simulink model "Modello_definitivo"  (Simulink 9.2)
settings: Solver=ode45  StartTime=0*24*3600  StopTime=365*24*3600  MaxStep=3600  RelTol=1e-3  SampleTimeConstraint=Specified  EnableMultiTasking=on
undefined symbols (not defined in the file or in its folder): T_s_in
libraries: simulink x1
(part 1 of 2)
settings Model: Creator=Matteo  LastModifiedBy=don-g
settings SolverCC: ZeroCrossControl=DisableAll
settings OptimizationCC: ExpressionDepthLimit=2147483647  InitFltsAndDblsToZero=on
settings DebuggingCC: SolverPrmCheckMsg=warning
settings SFSimCC: SimUseLocalCustomCode=on
settings RTWCC: RTWUseLocalCustomCode=on
settings GRTTargetCC: GeneratePreprocessorConditionals=Use local settings
settings ConfigComp: CovExternalEMLEnable=on

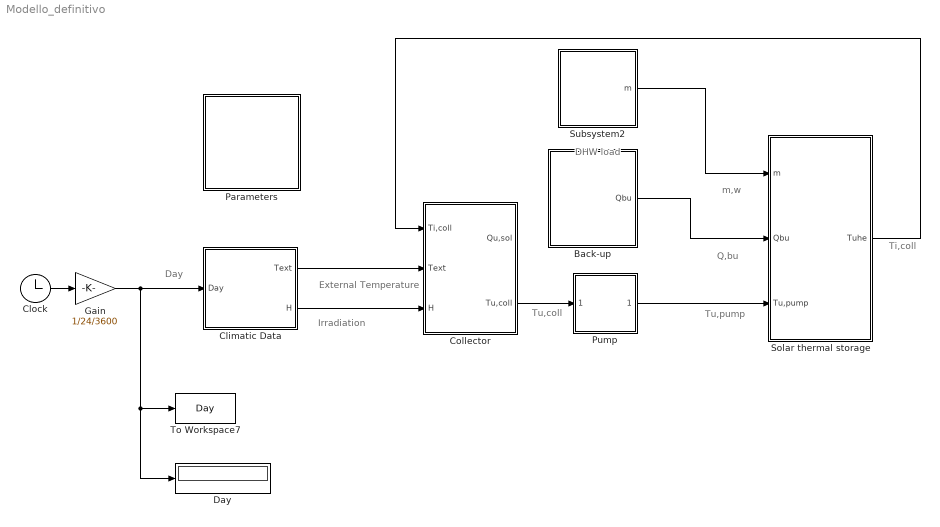
== system Modello_definitivo ==
  note: Q,bu
  note: m,w
  note: Day
  note: Irradiation
  note: External Temperature
  note: Tu,coll
  note: DHW load
  note: Tu,pump
  note: Ti,coll
  Back-up : Subsystem
      mask Display: image(imread('caldaia.jpg'))
  Climatic Data : Subsystem
      mask Display: image(imread('sole.jpg'))
  Clock : Clock
  Collector : Subsystem
      mask Display: image(imread('collettore.jpg'))
  Day : Display
  Gain : Gain  Gain=1/24/3600  SaturateOnIntegerOverflow=on  OutDataTypeStr=Inherit: Same as input  ParamDataTypeStr=Inherit: Same as input
  Parameters : Subsystem  mask{Gamma=0, Rho=0.2, Lat=44.48, Beta=0.01, Eta0=0.959, a1=8.91, a2=0.047, Nc=1, Aap=2.31, m_brine=0.010, Cp_brine=3900, L=1.7, Eta_pump=0.8, Eta_el=0.95, H_pressure=50000, Pump_power=65, Rho_brine=1037, T_room=20, BU_power=2000, Rho_water=1000, Cp_water=4186, U_s=1, T_s_in=45, D_s=0.6, V_s=168, H_s=0.99, UA_s_ex=167, T_s_max=90, A_s_ex=1.8, U_s_ex=1.1, T_DHW=45, S_u=200, T_acq=15}
      mask prompts: Gamma "Azimuth (°)"; Rho "Albedo"; Lat "Latitude (°)"; Beta "Tilt (°)"; Eta0 "Optical efficiency"; a1 "First order coefficient"; a2 "Second order coefficient"; Nc "Number of collectors"; Aap "Absorber area (m2)"; m_brine "Flow rate per surface area (kg/s*m2)"; Cp_brine "Cp brine (J/kgK)"; L "Collector liquid volume (lt)"; Eta_pump "Pump efficiency"; Eta_el "Electrical efficiency"; H_pressure "Head pressure (Pa)"; Pump_power "Pump power (W)"; Rho_brine "Brine density (kg/m3)"; T_room "Room temperature (°C)"; BU_power "Back-up power (W)"; Rho_water "Water density (kg/m3)"; Cp_water "Cp water (J/kgK)"; U_s "Storage U (W/m2K)"; T_s_in "Initial storage temperature (°C)"; D_s "Storage diameter (m)"; V_s "Storage volume (lt)"; H_s "Storage height (m)"; UA_s_ex "Solar exchanger UA (W/K)"; T_s_max "Maximum storage temperature (°C)"; A_s_ex "Heat exchanger area (m2)"; U_s_ex "U-value heat exchanger (W/m2K)"; T_DHW "DHW temperature (°C)"; S_u "Building energetic surface (m2)"; T_acq "Aqueduct temperature (°C)"
      mask Display: image(imread('images.jpg'))
  Pump : Subsystem
      mask Display: image(imread('pompa.jpg'))
  Solar thermal storage : Subsystem
      mask Display: image(imread('prova.jpg'))
  Subsystem2 : Subsystem
      mask Display: image(imread('casa.jpg'))
  To Workspace7 : ToWorkspace  VariableName=Day  SampleTime=[3600 0]
  wires:
  Gain/1 -> Climatic Data/1(Day), Day/1, To Workspace7/1
  Clock/1 -> Gain/1
  Climatic Data/1(Text) -> Collector/2(Text)
  Climatic Data/2(H) -> Collector/3(H)
  Collector/2(Tu,coll) -> Pump/1(Tu,coll)
  Subsystem2/1(m) -> Solar thermal storage/1(m)
  Pump/1(Tu,pump) -> Solar thermal storage/3(Tu,pump)
  Solar thermal storage/1(Tuhe) -> Collector/1(Ti,coll)
  Back-up/1(Qbu) -> Solar thermal storage/2(Qbu)

== system Modello_definitivo/Back-up ==
  Add1 : Sum  Inputs=-+
  Back-up energy [MJ] : Display
  Back-up energy [kWh] : Display
  Integral Block : Subsystem
  Product3 : Product  Inputs=**  SaturateOnIntegerOverflow=on  OutDataTypeStr=Inherit: Same as first input
  Prova back-up : Subsystem
  Relay : Relay  OnSwitchValue=0  OffSwitchValue=-5
  Scope2 : Scope
  To Workspace1 : ToWorkspace  VariableName=Ebu  SampleTime=[3600 0]
  To Workspace6 : ToWorkspace  VariableName=Qbu  SampleTime=[3600 0]
  Qbu : Outport
  tag scope: Ebu_kWh=global, Qbu=global
  wires:
  [T_DHW] -> Add1/2
  [T3] -> Add1/1
  Add1/1 -> Relay/1, Scope2/1
  Relay/1 -> Product3/2
  [BU_power] -> Product3/1
  Product3/1 -> Integral Block/1(Watt), [Qbu], To Workspace6/1, Qbu/1
  Integral Block/1(MJ) -> Back-up energy [MJ]/1
  Integral Block/2(kWh) -> [Ebu_kWh], Back-up energy [kWh]/1, To Workspace1/1

== system Modello_definitivo/Climatic Data ==
  Day : Inport
  Day Length [h] : Display
  From Workspace : FromWorkspace  VariableName=Irraggiamento_Globale_Wh  SampleTime=0
  From Workspace1 : FromWorkspace  VariableName=Temperature  SampleTime=0
  Mux4 : Mux  Inputs=2
  Scope16 : Scope
  Scope6 : Scope
  To Workspace2 : ToWorkspace  VariableName=Text  SampleTime=[3600 0]
  irraggiamento : Subsystem
  Text : Outport  SampleTime=[3600 0]
  H : Outport  Port=2
  tag scope: H=global
  wires:
  From Workspace1/1 -> Scope16/1, Text/1, To Workspace2/1
  From Workspace/1 -> Mux4/2, Scope6/1
  irraggiamento/2(Day Length) -> Day Length [h]/1
  irraggiamento/1(H) -> H/1, [H]
  Mux4/1 -> irraggiamento/1(Climatic Data Input)
  Day/1 -> Mux4/1

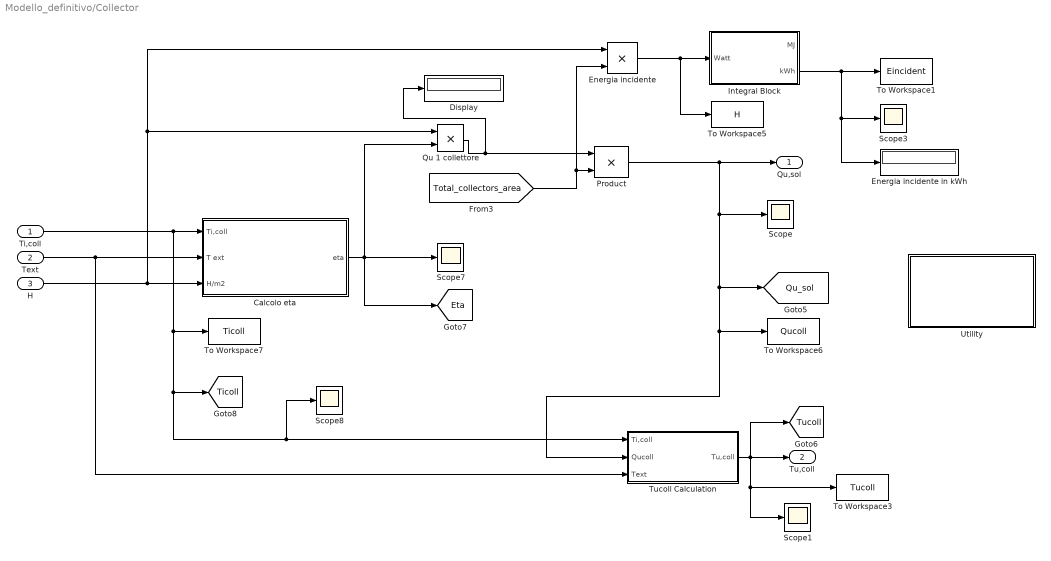
== system Modello_definitivo/Collector ==
  Ti,coll : Inport
  Text : Inport  Port=2
  H : Inport  Port=3
  Calcolo eta : Subsystem
  Display : Display
  Energia incidente : Product  RndMeth=Zero
  Energia incidente in kWh : Display
  Integral Block : Subsystem
  Product : Product  RndMeth=Zero
  Qu 1 collettore : Product  RndMeth=Zero
  Scope{,1,3,7..8} (5 alike) : Scope
  To Workspace1 : ToWorkspace  VariableName=Eincident  SampleTime=[3600 0]
  To Workspace3 : ToWorkspace  VariableName=Tucoll  SampleTime=[3600 0]
  To Workspace5 : ToWorkspace  VariableName=H  SampleTime=[3600 0]
  To Workspace6 : ToWorkspace  VariableName=Qucoll  SampleTime=[3600 0]
  To Workspace7 : ToWorkspace  VariableName=Ticoll  SampleTime=[3600 0]
  Tucoll Calculation : Subsystem
  Utility : Subsystem
  Qu,sol : Outport
  Tu,coll : Outport  Port=2
  tag scope: Eta=global, Qu_sol=global, Ticoll=global, Tucoll=global
  wires:
  H/1 -> Calcolo eta/3(H/m2), Qu 1 collettore/1, Energia incidente/1
  Text/1 -> Calcolo eta/2(T ext), Tucoll Calculation/3(Text)
  Calcolo eta/1(eta) -> [Eta], Qu 1 collettore/2, Scope7/1
  Qu 1 collettore/1 -> Product/1, Display/1
  Tucoll Calculation/1(Tu,coll) -> Tu,coll/1, Scope1/1, To Workspace3/1, [Tucoll]
  Energia incidente/1 -> Integral Block/1(Watt), To Workspace5/1
  Product/1 -> Qu,sol/1, [Qu_sol], To Workspace6/1, Tucoll Calculation/2(Qucoll), Scope/1
  Ti,coll/1 -> [Ticoll], Tucoll Calculation/1(Ti,coll), Scope8/1, To Workspace7/1, Calcolo eta/1(Ti,coll)
  Integral Block/2(kWh) -> To Workspace1/1, Scope3/1, Energia incidente in kWh/1
  [Total_collectors_area] -> Product/2, Energia incidente/2

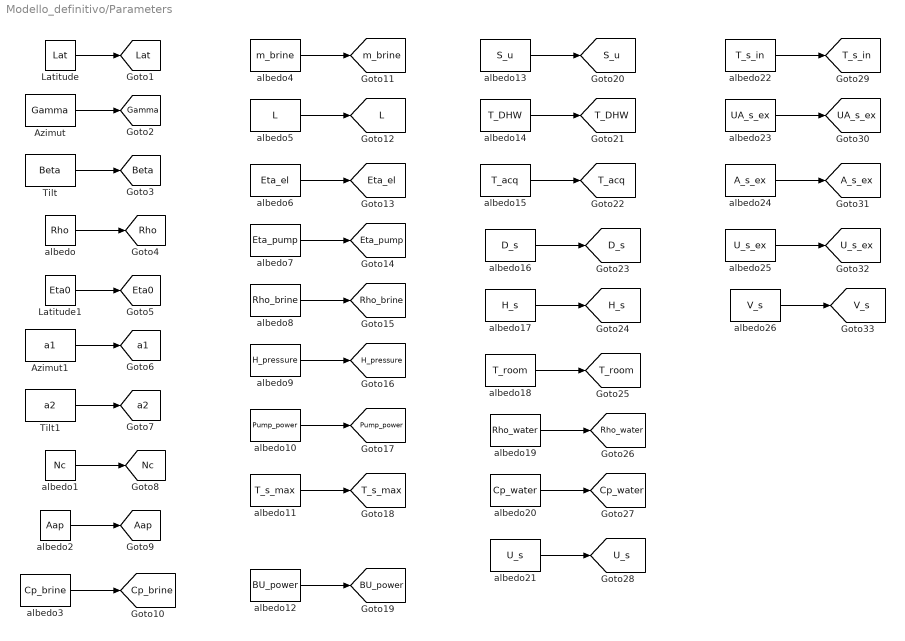
== system Modello_definitivo/Parameters ==
  Azimut : Constant  Value=Gamma
  Azimut1 : Constant  Value=a1
  Latitude : Constant  Value=Lat
  Latitude1 : Constant  Value=Eta0
  Tilt : Constant  Value=Beta
  Tilt1 : Constant  Value=a2
  albedo : Constant  Value=Rho
  albedo1 : Constant  Value=Nc
  albedo10 : Constant  Value=Pump_power
  albedo11 : Constant  Value=T_s_max
  albedo12 : Constant  Value=BU_power
  albedo13 : Constant  Value=S_u
  albedo14 : Constant  Value=T_DHW
  albedo15 : Constant  Value=T_acq
  albedo16 : Constant  Value=D_s
  albedo17 : Constant  Value=H_s
  albedo18 : Constant  Value=T_room
  albedo19 : Constant  Value=Rho_water
  albedo2 : Constant  Value=Aap
  albedo20 : Constant  Value=Cp_water
  albedo21 : Constant  Value=U_s
  albedo22 : Constant  Value=T_s_in
  albedo23 : Constant  Value=UA_s_ex
  albedo24 : Constant  Value=A_s_ex
  albedo25 : Constant  Value=U_s_ex
  albedo26 : Constant  Value=V_s
  albedo3 : Constant  Value=Cp_brine
  albedo4 : Constant  Value=m_brine
  albedo5 : Constant  Value=L
  albedo6 : Constant  Value=Eta_el
  albedo7 : Constant  Value=Eta_pump
  albedo8 : Constant  Value=Rho_brine
  albedo9 : Constant  Value=H_pressure
  tag scope: A_s_ex=global, Aap=global, BU_power=global, Beta=global, Cp_brine=global, Cp_water=global, D_s=global, Eta0=global, Eta_el=global, Eta_pump=global, Gamma=global, H_pressure=global, H_s=global, L=global, Lat=global, Nc=global, Pump_power=global, Rho=global, Rho_brine=global, Rho_water=global, S_u=global, T_DHW=global, T_acq=global, T_room=global, T_s_in=global, T_s_max=global, UA_s_ex=global, U_s=global, U_s_ex=global, V_s=global, a1=global, a2=global, m_brine=global
  wires:
  Latitude/1 -> [Lat]
  Azimut/1 -> [Gamma]
  Tilt/1 -> [Beta]
  albedo/1 -> [Rho]
  Latitude1/1 -> [Eta0]
  Azimut1/1 -> [a1]
  Tilt1/1 -> [a2]
  albedo1/1 -> [Nc]
  albedo2/1 -> [Aap]
  albedo3/1 -> [Cp_brine]
  albedo4/1 -> [m_brine]
  albedo5/1 -> [L]
  albedo6/1 -> [Eta_el]
  albedo7/1 -> [Eta_pump]
  albedo8/1 -> [Rho_brine]
  albedo9/1 -> [H_pressure]
  albedo10/1 -> [Pump_power]
  albedo11/1 -> [T_s_max]
  albedo12/1 -> [BU_power]
  albedo13/1 -> [S_u]
  albedo14/1 -> [T_DHW]
  albedo15/1 -> [T_acq]
  albedo16/1 -> [D_s]
  albedo17/1 -> [H_s]
  albedo18/1 -> [T_room]
  albedo19/1 -> [Rho_water]
  albedo20/1 -> [Cp_water]
  albedo21/1 -> [U_s]
  albedo22/1 -> [T_s_in]
  albedo23/1 -> [UA_s_ex]
  albedo24/1 -> [A_s_ex]
  albedo25/1 -> [U_s_ex]
  albedo26/1 -> [V_s]

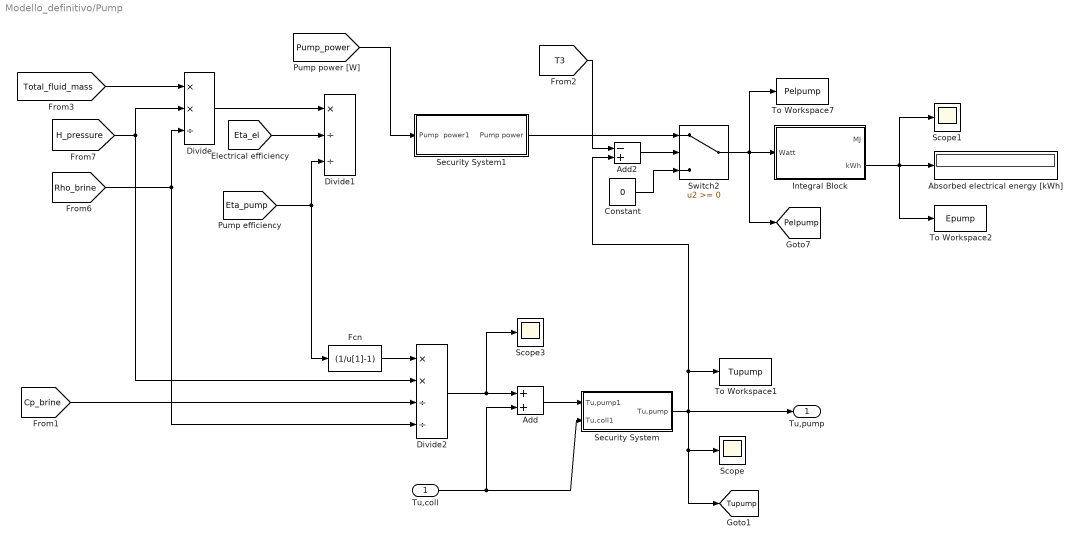
== system Modello_definitivo/Pump ==
  Tu,coll : Inport
  Absorbed electrical energy [kWh] : Display
  Add : Sum
  Add2 : Sum  Inputs=-+
  Constant : Constant  Value=0
  Divide : Product  Inputs=**/
  Divide1 : Product  Inputs=*//
  Divide2 : Product  Inputs=**//
  Fcn : Fcn  Expr=(1/u[1]-1)
  Integral Block : Subsystem
  Scope : Scope
  Scope1 : Scope
  Scope3 : Scope
  Security System : Subsystem
  Security System1 : Subsystem
  Switch2 : Switch  ZeroCross=off
  To Workspace1 : ToWorkspace  VariableName=Tupump  SampleTime=[3600 0]
  To Workspace2 : ToWorkspace  VariableName=Epump  SampleTime=[3600 0]
  To Workspace7 : ToWorkspace  VariableName=Pelpump  SampleTime=[3600 0]
  Tu,pump : Outport
  tag scope: Pelpump=global, Tupump=global
  wires:
  [Total_fluid_mass] -> Divide/1
  [H_pressure] -> Divide/2, Divide2/2
  [Rho_brine] -> Divide/3, Divide2/4
  Divide/1 -> Divide1/1
  [Eta_pump] -> Fcn/1, Divide1/3
  Fcn/1 -> Divide2/1
  Divide2/1 -> Add/1, Scope3/1
  Tu,coll/1 -> Security System/2(Tu,coll1), Add/2
  [Cp_brine] -> Divide2/3
  Integral Block/2(kWh) -> Absorbed electrical energy [kWh]/1, Scope1/1, To Workspace2/1
  Add/1 -> Security System/1(Tu,pump1)
  Security System/1(Tu,pump) -> To Workspace1/1, Add2/2, Scope/1, [Tupump], Tu,pump/1
  [Eta_el] -> Divide1/2
  [Pump_power] -> Security System1/1(Pump  power1)
  Security System1/1(Pump power) -> Switch2/1
  Add2/1 -> Switch2/2
  [T3] -> Add2/1
  Switch2/1 -> To Workspace7/1, [Pelpump], Integral Block/1(Watt)
  Constant/1 -> Switch2/3

== system Modello_definitivo/Solar thermal storage ==
  note: V[m3]
  m : Inport
  Qbu : Inport  Port=2
  Tu,pump : Inport  Port=3
  Divide : Product  Inputs=*/
  Lower part 3 : Subsystem
  Tuhe : Outport
  tag scope: m=global
  wires:
  [V_s] -> Divide/1
  Divide/1 -> Lower part 3/1(V)
  [Rho_water] -> Divide/2
  Lower part 3/2(Tuhe) -> Tuhe/1
  Tu,pump/1 -> Lower part 3/2(Tupump)
  Qbu/1 -> Lower part 3/3(Qbu)
  m/1 -> [m]

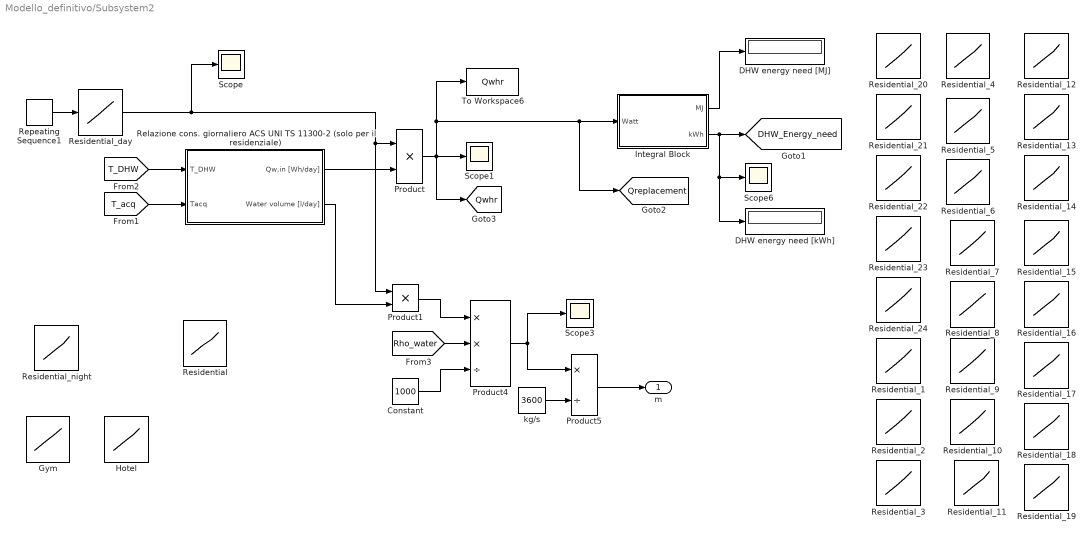
== system Modello_definitivo/Subsystem2 ==
  Constant : Constant  Value=1000
  DHW energy need [MJ] : Display
      settings: Format=bank
  DHW energy need [kWh] : Display
  Gym : Lookup  InputValues=[0*3600 1*3600 2*3600 3*3600 4*3600 5*3600 6*3600 7*3600 8*3600 9*3600 10*3600 11*3600 12*3600 13*3600 14*3600 15*3600 16*3600 17*3600 18*3600 19*3600 20*3600 21*3600 22*3600 23*3600 24*3600]  Table=[0.028 0 0 0 0 0 0 0 0.007 0.025 0.025 0.028 0.139 0.139 0.139 0.028 0.028 0.028 0.139 0.139 0.028 0.139 0.0139 0.0139 0.028]  SaturateOnIntegerOverflow=on
  Hotel : Lookup  InputValues=[0*3600 6.5*3600 6.5*3600 9.5*3600 9.5*3600 18.5*3600 18.5*3600 21*3600 21*3600 24*3600]  SaturateOnIntegerOverflow=on
  Integral Block : Subsystem
  Product : Product  SaturateOnIntegerOverflow=on  OutDataTypeStr=Inherit: Same as first input
  Product1 : Product  SaturateOnIntegerOverflow=on  OutDataTypeStr=Inherit: Same as first input
  Product4 : Product  Inputs=**/  SaturateOnIntegerOverflow=on  OutDataTypeStr=Inherit: Same as first input
  Product5 : Product  Inputs=*/  SaturateOnIntegerOverflow=on  OutDataTypeStr=Inherit: Same as first input
  Relazione cons. giornaliero ACS UNI TS 11300-2 (solo per il residenziale) : Subsystem
  Repeating Sequence1 : simulink/Sources/Repeating Sequence  rep_seq_t=[0 24*3600]  rep_seq_y=[0 24*3600]
  Residential : Lookup  InputValues=[0*3600 1*3600 2*3600 3*3600 4*3600 5*3600 6*3600 7*3600 8*3600 9*3600 10*3600 11*3600 12*3600 13*3600 14*3600 15*3600 16*3600 17*3600 18*3600 19*3600 20*3600 21*3600 22*3600 23*3600 24*3600]  Table=[0 0.025 0.028 0.028 0 0 0 0.139 0.139 0.139 0.028 0.028 0.028 0.028 0.007 0.007 0.007 0.007 0.139 0.139 0.028 0.028 0.028 0 0]  SaturateOnIntegerOverflow=on
  Residential_1 : Lookup  InputValues=[0,3600,7200,10800,14400,18000,21600,25200,28800,32400,36000,39600,43200,46800,50400,54000,57600,61200,64800,68400,72000,75600,79200,82800,86400]  Table=[0.2,0.2,0.2,0,0,0,0,0,0,0,0,0,0,0,0,0,0,0,0,0,0,0,0.2,0.2,0.2]  SaturateOnIntegerOverflow=on
  Residential_10 : Lookup  InputValues=[0,3600,7200,10800,14400,18000,21600,25200,28800,32400,36000,39600,43200,46800,50400,54000,57600,61200,64800,68400,72000,75600,79200,82800,86400]  Table=[0,0,0,0,0,0,0,0.2,0.2,0.2,0.2,0.2,0,0,0,0,0,0,0,0,0,0,0,0,0]  SaturateOnIntegerOverflow=on
  Residential_11 : Lookup  InputValues=[0,3600,7200,10800,14400,18000,21600,25200,28800,32400,36000,39600,43200,46800,50400,54000,57600,61200,64800,68400,72000,75600,79200,82800,86400]  Table=[0,0,0,0,0,0,0,0,0.2,0.2,0.2,0.2,0.2,0,0,0,0,0,0,0,0,0,0,0,0]  SaturateOnIntegerOverflow=on
  Residential_12 : Lookup  InputValues=[0,3600,7200,10800,14400,18000,21600,25200,28800,32400,36000,39600,43200,46800,50400,54000,57600,61200,64800,68400,72000,75600,79200,82800,86400]  Table=[0,0,0,0,0,0,0,0,0,0.2,0.2,0.2,0.2,0.2,0,0,0,0,0,0,0,0,0,0,0]  SaturateOnIntegerOverflow=on
  Residential_13 : Lookup  InputValues=[0,3600,7200,10800,14400,18000,21600,25200,28800,32400,36000,39600,43200,46800,50400,54000,57600,61200,64800,68400,72000,75600,79200,82800,86400]  Table=[0,0,0,0,0,0,0,0,0,0,0.2,0.2,0.2,0.2,0.2,0,0,0,0,0,0,0,0,0,0]  SaturateOnIntegerOverflow=on
  Residential_14 : Lookup  InputValues=[0,3600,7200,10800,14400,18000,21600,25200,28800,32400,36000,39600,43200,46800,50400,54000,57600,61200,64800,68400,72000,75600,79200,82800,86400]  Table=[0,0,0,0,0,0,0,0,0,0,0,0.2,0.2,0.2,0.2,0.2,0,0,0,0,0,0,0,0,0]  SaturateOnIntegerOverflow=on
  Residential_15 : Lookup  InputValues=[0,3600,7200,10800,14400,18000,21600,25200,28800,32400,36000,39600,43200,46800,50400,54000,57600,61200,64800,68400,72000,75600,79200,82800,86400]  Table=[0,0,0,0,0,0,0,0,0,0,0,0,0.2,0.2,0.2,0.2,0.2,0,0,0,0,0,0,0,0]  SaturateOnIntegerOverflow=on
  Residential_16 : Lookup  InputValues=[0,3600,7200,10800,14400,18000,21600,25200,28800,32400,36000,39600,43200,46800,50400,54000,57600,61200,64800,68400,72000,75600,79200,82800,86400]  Table=[0,0,0,0,0,0,0,0,0,0,0,0,0,0.2,0.2,0.2,0.2,0.2,0,0,0,0,0,0,0]  SaturateOnIntegerOverflow=on
  Residential_17 : Lookup  InputValues=[0,3600,7200,10800,14400,18000,21600,25200,28800,32400,36000,39600,43200,46800,50400,54000,57600,61200,64800,68400,72000,75600,79200,82800,86400]  Table=[0,0,0,0,0,0,0,0,0,0,0,0,0,0,0.2,0.2,0.2,0.2,0.2,0,0,0,0,0,0]  SaturateOnIntegerOverflow=on
  Residential_18 : Lookup  InputValues=[0,3600,7200,10800,14400,18000,21600,25200,28800,32400,36000,39600,43200,46800,50400,54000,57600,61200,64800,68400,72000,75600,79200,82800,86400]  Table=[0,0,0,0,0,0,0,0,0,0,0,0,0,0,0,0.2,0.2,0.2,0.2,0.2,0,0,0,0,0]  SaturateOnIntegerOverflow=on
  Residential_19 : Lookup  InputValues=[0,3600,7200,10800,14400,18000,21600,25200,28800,32400,36000,39600,43200,46800,50400,54000,57600,61200,64800,68400,72000,75600,79200,82800,86400]  Table=[0,0,0,0,0,0,0,0,0,0,0,0,0,0,0,0,0.2,0.2,0.2,0.2,0.2,0,0,0,0]  SaturateOnIntegerOverflow=on
  Residential_2 : Lookup  InputValues=[0,3600,7200,10800,14400,18000,21600,25200,28800,32400,36000,39600,43200,46800,50400,54000,57600,61200,64800,68400,72000,75600,79200,82800,86400]  Table=[0.2,0.2,0.2,0.2,0,0,0,0,0,0,0,0,0,0,0,0,0,0,0,0,0,0,0,0.2,0.2]  SaturateOnIntegerOverflow=on
  Residential_20 : Lookup  InputValues=[0,3600,7200,10800,14400,18000,21600,25200,28800,32400,36000,39600,43200,46800,50400,54000,57600,61200,64800,68400,72000,75600,79200,82800,86400]  Table=[0,0,0,0,0,0,0,0,0,0,0,0,0,0,0,0,0,0.2,0.2,0.2,0.2,0.2,0,0,0]  SaturateOnIntegerOverflow=on
  Residential_21 : Lookup  InputValues=[0,3600,7200,10800,14400,18000,21600,25200,28800,32400,36000,39600,43200,46800,50400,54000,57600,61200,64800,68400,72000,75600,79200,82800,86400]  Table=[0,0,0,0,0,0,0,0,0,0,0,0,0,0,0,0,0,0,0.2,0.2,0.2,0.2,0.2,0,0]  SaturateOnIntegerOverflow=on
  Residential_22 : Lookup  InputValues=[0,3600,7200,10800,14400,18000,21600,25200,28800,32400,36000,39600,43200,46800,50400,54000,57600,61200,64800,68400,72000,75600,79200,82800,86400]  Table=[0,0,0,0,0,0,0,0,0,0,0,0,0,0,0,0,0,0,0,0.2,0.2,0.2,0.2,0.2,0]  SaturateOnIntegerOverflow=on
  Residential_23 : Lookup  InputValues=[0,3600,7200,10800,14400,18000,21600,25200,28800,32400,36000,39600,43200,46800,50400,54000,57600,61200,64800,68400,72000,75600,79200,82800,86400]  Table=[0.2,0,0,0,0,0,0,0,0,0,0,0,0,0,0,0,0,0,0,0,0.2,0.2,0.2,0.2,0.2]  SaturateOnIntegerOverflow=on
  Residential_24 : Lookup  InputValues=[0,3600,7200,10800,14400,18000,21600,25200,28800,32400,36000,39600,43200,46800,50400,54000,57600,61200,64800,68400,72000,75600,79200,82800,86400]  Table=[0.2,0.2,0,0,0,0,0,0,0,0,0,0,0,0,0,0,0,0,0,0,0,0.2,0.2,0.2,0.2]  SaturateOnIntegerOverflow=on
  Residential_3 : Lookup  InputValues=[0,3600,7200,10800,14400,18000,21600,25200,28800,32400,36000,39600,43200,46800,50400,54000,57600,61200,64800,68400,72000,75600,79200,82800,86400]  Table=[0.2,0.2,0.2,0.2,0.2,0,0,0,0,0,0,0,0,0,0,0,0,0,0,0,0,0,0,0,0.2]  SaturateOnIntegerOverflow=on
  Residential_4 : Lookup  InputValues=[0,3600,7200,10800,14400,18000,21600,25200,28800,32400,36000,39600,43200,46800,50400,54000,57600,61200,64800,68400,72000,75600,79200,82800,86400]  Table=[0,0.2,0.2,0.2,0.2,0.2,0,0,0,0,0,0,0,0,0,0,0,0,0,0,0,0,0,0,0]  SaturateOnIntegerOverflow=on
  Residential_5 : Lookup  InputValues=[0,3600,7200,10800,14400,18000,21600,25200,28800,32400,36000,39600,43200,46800,50400,54000,57600,61200,64800,68400,72000,75600,79200,82800,86400]  Table=[0,0,0.2,0.2,0.2,0.2,0.2,0,0,0,0,0,0,0,0,0,0,0,0,0,0,0,0,0,0]  SaturateOnIntegerOverflow=on
  Residential_6 : Lookup  InputValues=[0,3600,7200,10800,14400,18000,21600,25200,28800,32400,36000,39600,43200,46800,50400,54000,57600,61200,64800,68400,72000,75600,79200,82800,86400]  Table=[0,0,0,0.2,0.2,0.2,0.2,0.2,0,0,0,0,0,0,0,0,0,0,0,0,0,0,0,0,0]  SaturateOnIntegerOverflow=on
  Residential_7 : Lookup  InputValues=[0,3600,7200,10800,14400,18000,21600,25200,28800,32400,36000,39600,43200,46800,50400,54000,57600,61200,64800,68400,72000,75600,79200,82800,86400]  Table=[0,0,0,0,0.2,0.2,0.2,0.2,0.2,0,0,0,0,0,0,0,0,0,0,0,0,0,0,0,0]  SaturateOnIntegerOverflow=on
  Residential_8 : Lookup  InputValues=[0,3600,7200,10800,14400,18000,21600,25200,28800,32400,36000,39600,43200,46800,50400,54000,57600,61200,64800,68400,72000,75600,79200,82800,86400]  Table=[0,0,0,0,0,0.2,0.2,0.2,0.2,0.2,0,0,0,0,0,0,0,0,0,0,0,0,0,0,0]  SaturateOnIntegerOverflow=on
  Residential_9 : Lookup  InputValues=[0,3600,7200,10800,14400,18000,21600,25200,28800,32400,36000,39600,43200,46800,50400,54000,57600,61200,64800,68400,72000,75600,79200,82800,86400]  Table=[0,0,0,0,0,0,0.2,0.2,0.2,0.2,0.2,0,0,0,0,0,0,0,0,0,0,0,0,0,0]  SaturateOnIntegerOverflow=on
  Residential_day : Lookup  InputValues=[0,3600,7200,10800,14400,18000,21600,25200,28800,32400,36000,39600,43200,46800,50400,54000,57600,61200,64800,68400,72000,75600,79200,82800,86400]  Table=[0,0,0,0,0,0,0.0769,0.0769,0.0769,0.0769,0.0769,0.0769,0.0769,0.0769,0.0769,0.0769,0.0769,0.0769,0.0769,0,0,0,0,0,0]  SaturateOnIntegerOverflow=on
  Residential_night : Lookup  InputValues=[0,3600,7200,10800,14400,18000,21600,25200,28800,32400,36000,39600,43200,46800,50400,54000,57600,61200,64800,68400,72000,75600,79200,82800,86400]  Table=[0.143,0.143,0.143,0.143,0.143,0,0,0,0,0,0,0,0,0,0,0,0,0,0,0,0,0,0.143,0.143,0.143]  SaturateOnIntegerOverflow=on
  Scope{,1,3,6} (4 alike) : Scope
  To Workspace6 : ToWorkspace  VariableName=Qwhr  SampleTime=[3600 0]
  kg/s : Constant  Value=3600
  m : Outport
  tag scope: DHW_Energy_need=global, Qreplacement=global, Qwhr=global
  wires:
  Repeating Sequence1/1 -> Residential_day/1
  Product/1 -> Scope1/1, [Qwhr], To Workspace6/1, Integral Block/1(Watt), [Qreplacement]
  [T_DHW] -> Relazione cons. giornaliero ACS UNI TS 11300-2 (solo per il residenziale)/1(T_DHW)
  Residential_day/1 -> Scope/1, Product1/1, Product/1
  Relazione cons. giornaliero ACS UNI TS 11300-2 (solo per il residenziale)/1(Qw,in [Wh/day]) -> Product/2
  Relazione cons. giornaliero ACS UNI TS 11300-2 (solo per il residenziale)/2(Water volume [l/day]) -> Product1/2
  ? -> ?
  [T_acq] -> Relazione cons. giornaliero ACS UNI TS 11300-2 (solo per il residenziale)/2(Tacq)
  Product1/1 -> Product4/1
  [Rho_water] -> Product4/2
  Constant/1 -> Product4/3
  Product4/1 -> Scope3/1, Product5/1
  kg/s/1 -> Product5/2
  Product5/1 -> m/1
  Integral Block/1(MJ) -> DHW energy need [MJ]/1
  Integral Block/2(kWh) -> [DHW_Energy_need], Scope6/1, DHW energy need [kWh]/1

== system Modello_definitivo/Back-up/Integral Block ==
  Watt : Inport
  Integrator : Integrator
  J to MJ : Gain  Gain=1/1000000
  MJ to kWh : Gain  Gain=1/3.6
  MJ1 : Display
  Scope1 : Scope
  Scope2 : Scope
  kWh1 : Display
  MJ : Outport
  kWh : Outport  Port=2
  wires:
  Integrator/1 -> J to MJ/1
  Watt/1 -> Integrator/1
  J to MJ/1 -> Scope1/1, MJ1/1, MJ/1, MJ to kWh/1
  MJ to kWh/1 -> Scope2/1, kWh1/1, kWh/1

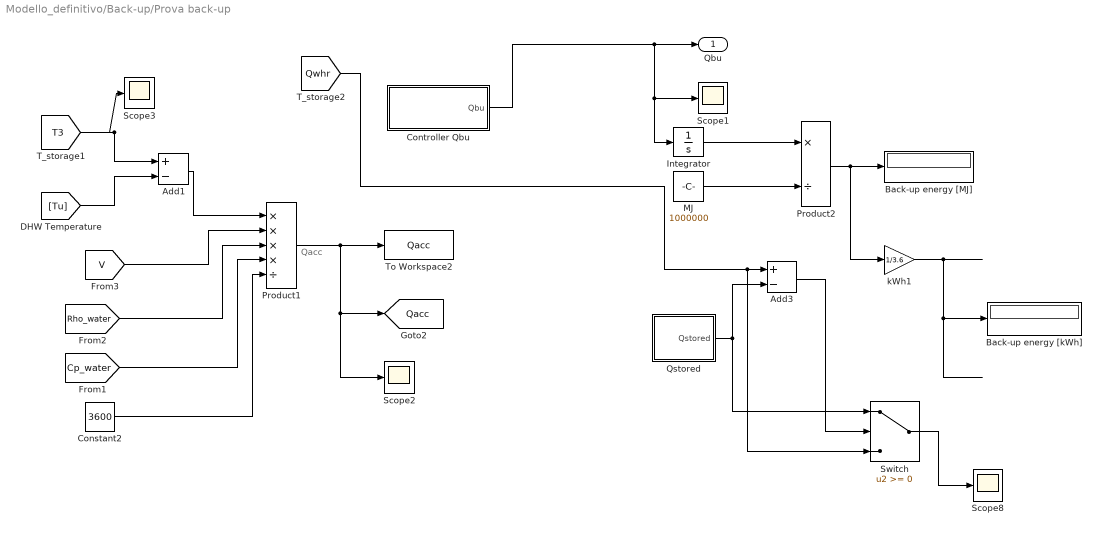
== system Modello_definitivo/Back-up/Prova back-up ==
  note: Qacc
  Add1 : Sum  Inputs=+-
  Add3 : Sum  Inputs=+-
  Back-up energy [MJ] : Display
  Back-up energy [kWh] : Display
  Constant2 : Constant  Value=3600
  Controller Qbu : Subsystem
  Integrator : Integrator
  MJ : Constant  Value=1000000
  Product1 : Product  Inputs=****/  SaturateOnIntegerOverflow=on  OutDataTypeStr=Inherit: Same as first input
  Product2 : Product  Inputs=*/  SaturateOnIntegerOverflow=on  OutDataTypeStr=Inherit: Same as first input
  Qstored : Subsystem
  Scope{1..3,8} (4 alike) : Scope
  Switch : Switch  ZeroCross=off
  To Workspace2 : ToWorkspace  VariableName=Qacc  SampleTime=[3600 0]
  kWh1 : Gain  Gain=1/3.6
  Qbu : Outport
  tag scope: Qacc=global
  wires:
  [Tu] -> Add1/2
  [T3] -> Add1/1, Scope3/1
  Integrator/1 -> Product2/1
  MJ/1 -> Product2/2
  Product2/1 -> Back-up energy [MJ]/1, kWh1/1
  kWh1/1 -> Back-up energy [kWh]/1
  Add1/1 -> Product1/1
  [V] -> Product1/2
  [Rho_water] -> Product1/3
  Product1/1 -> To Workspace2/1, Scope2/1, [Qacc]
  [Cp_water] -> Product1/4
  Constant2/1 -> Product1/5
  [Qwhr] -> Add3/1, Switch/3
  Controller Qbu/1(Qbu) -> Qbu/1, Scope1/1, Integrator/1
  Switch/1 -> Scope8/1
  Qstored/1(Qstored) -> Add3/2, Switch/1
  Add3/1 -> Switch/2

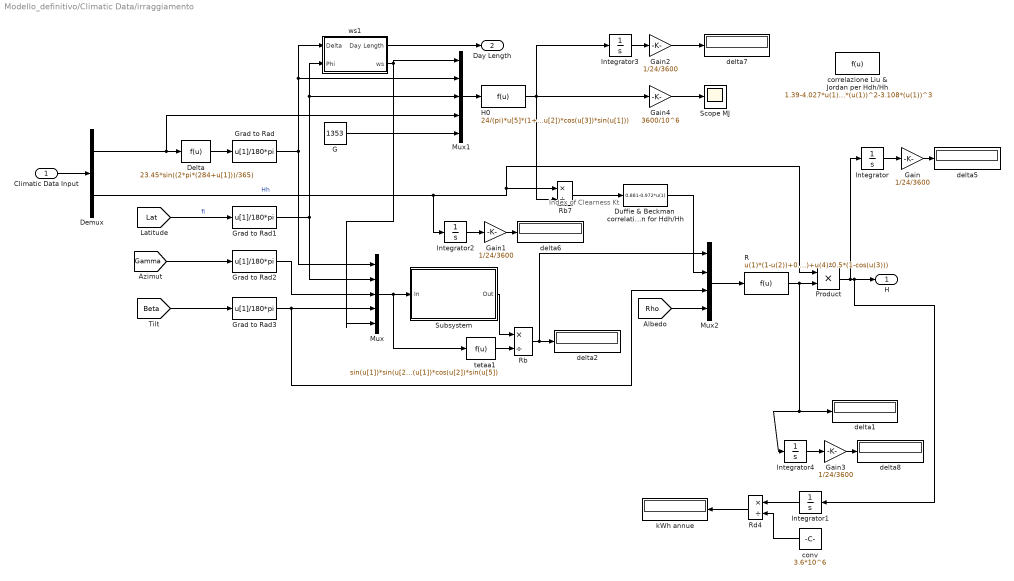
== system Modello_definitivo/Climatic Data/irraggiamento ==
  note: Index of Clearness Kt
  Climatic Data Input : Inport
  Delta : Fcn  Expr=23.45*sin((2*pi*(284+u[1]))/365)
  Demux : Demux  Outputs=2
  Duffie & Beckman  correlation for Hdh/Hh : Fcn  Expr=0.881-0.972*u(1)
  G : Constant  Value=1353
  Gain{,1..3} (4 alike) : Gain  Gain=1/24/3600
  Gain4 : Gain  Gain=3600/10^6
  Grad to Rad{,1..3} (4 alike) : Fcn  Expr=u[1]/180*pi
  H0 : Fcn  Expr=24/(pi)*u[5]*(1+0.033*cos((2*pi*u[4])/365))*(sin(u[2])*sin(u[3])*u(1)+cos(u[2])*cos(u[3])*sin(u[1]))
  Integrator{,1..4} (5 alike) : Integrator
  Mux : Mux  Inputs=5
  Mux1 : Mux  Inputs=5
  Mux2 : Mux
  Product : Product  RndMeth=Zero
  R : Fcn  Expr=u(1)*(1-u(2))+0.5*(1+cos(u(3)))*u(2)+u(4)*0.5*(1-cos(u(3)))
  Rb : Product  Inputs=*/  SaturateOnIntegerOverflow=on  OutDataTypeStr=Inherit: Same as first input
  Rb7 : Product  Inputs=*/  SaturateOnIntegerOverflow=on  OutDataTypeStr=Inherit: Same as first input
  Rd4 : Product  Inputs=*/  SaturateOnIntegerOverflow=on  OutDataTypeStr=Inherit: Same as first input
  Scope MJ : Scope
  Subsystem : Subsystem
  conv : Constant  Value=3.6*10^6
  correlazione Liu & Jordan per Hdh/Hh : Fcn  Expr=1.39-4.027*u(1)+5.531*(u(1))^2-3.108*(u(1))^3
  delta{1..2,5..8} (6 alike) : Display
  kWh annue : Display
  tetaa1 : Fcn  Expr=sin(u[1])*sin(u[2])*u(5)+cos(u[1])*cos(u[2])*sin(u[5])
  ws1 : Subsystem
  H : Outport  SampleTime=[3600 0]
  Day Length : Outport  Port=2
  wires:
  Grad to Rad/1 -> ws1/1(Delta), Mux1/2, Mux/1
  Delta/1 -> Grad to Rad/1
  Mux1/1 -> H0/1
  H0/1 -> Integrator3/1, Gain4/1, Rb7/2
  ws1/2(ws) -> Mux1/1, Mux/5
  Climatic Data Input/1 -> Demux/1
  [Lat] -> Grad to Rad1/1  "fi"
  G/1 -> Mux1/5
  Demux/2 -> Integrator2/1, Rb7/1, Product/1  "Hh"
  Rb7/1 -> Duffie & Beckman  correlation for Hdh/Hh/1
  Mux/1 -> tetaa1/1, Subsystem/1(In)
  tetaa1/1 -> Rb/2
  Rb/1 -> delta2/1, Mux2/1
  Mux2/1 -> R/1
  [Rho] -> Mux2/4
  Duffie & Beckman  correlation for Hdh/Hh/1 -> Mux2/2
  R/1 -> delta1/1, Integrator4/1, Product/2
  Product/1 -> H/1, Integrator1/1, Integrator/1
  Subsystem/1(Out) -> Rb/1
  Grad to Rad1/1 -> Mux1/3, ws1/2(Phi), Mux/2
  [Gamma] -> Grad to Rad2/1
  Demux/1 -> Delta/1, Mux1/4
  Grad to Rad2/1 -> Mux/3
  [Beta] -> Grad to Rad3/1
  Grad to Rad3/1 -> Mux2/3, Mux/4
  Integrator/1 -> Gain/1
  Gain/1 -> delta5/1
  Integrator1/1 -> Rd4/1
  Rd4/1 -> kWh annue/1
  conv/1 -> Rd4/2
  Integrator2/1 -> Gain1/1
  Gain1/1 -> delta6/1
  Integrator3/1 -> Gain2/1
  Gain2/1 -> delta7/1
  Integrator4/1 -> Gain3/1
  Gain3/1 -> delta8/1
  Gain4/1 -> Scope MJ/1
  ws1/1(Day Length) -> Day Length/1

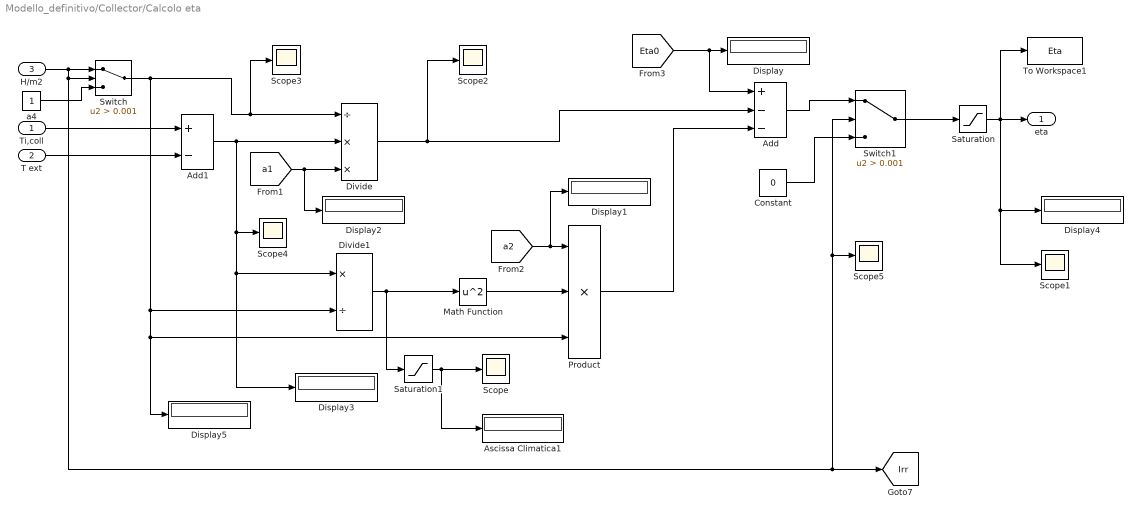
== system Modello_definitivo/Collector/Calcolo eta ==
  Ti,coll : Inport
  T ext : Inport  Port=2
  H/m2 : Inport  Port=3
  Add : Sum  Inputs=+--
  Add1 : Sum  Inputs=+-
  Ascissa Climatica1 : Display
  Constant : Constant  Value=0
  Display{,1..5} (6 alike) : Display
  Divide : Product  Inputs=/**
  Divide1 : Product  Inputs=*/
  Math Function : Math  Operator=square  SaturateOnIntegerOverflow=on
  Product : Product  Inputs=3  RndMeth=Zero
  Saturation : Saturate  UpperLimit=1  LowerLimit=-inf
  Saturation1 : Saturate  UpperLimit=1  LowerLimit=0
  Scope{,1..5} (6 alike) : Scope
  Switch : Switch  Criteria=u2 > Threshold  Threshold=0.001  ZeroCross=off
  Switch1 : Switch  Criteria=u2 > Threshold  Threshold=0.001
  To Workspace1 : ToWorkspace  VariableName=Eta  SampleTime=[3600 0]
  a4 : Constant
  eta : Outport
  tag scope: Irr=global
  wires:
  Add1/1 -> Divide/2, Scope4/1, Display3/1, Divide1/1
  [a1] -> Display2/1, Divide/3
  Divide1/1 -> Saturation1/1, Math Function/1
  [a2] -> Product/1, Display1/1
  Math Function/1 -> Product/2
  [Eta0] -> Add/1, Display/1
  Divide/1 -> Add/2, Scope2/1
  Product/1 -> Add/3
  Saturation/1 -> eta/1, Display4/1, Scope1/1, To Workspace1/1
  T ext/1 -> Add1/2
  Ti,coll/1 -> Add1/1
  H/m2/1 -> Switch/1, Switch/2, Switch1/2, Scope5/1, [Irr]
  Switch/1 -> Divide/1, Scope3/1, Display5/1, Product/3, Divide1/2
  Add/1 -> Switch1/1
  Constant/1 -> Switch1/3
  Switch1/1 -> Saturation/1
  Saturation1/1 -> Scope/1, Ascissa Climatica1/1
  a4/1 -> Switch/3

== system Modello_definitivo/Collector/Integral Block ==
  Watt : Inport
  Integrator : Integrator
  J to MJ : Gain  Gain=1/1000000
  MJ to kWh : Gain  Gain=1/3.6
  MJ1 : Display
  Scope1 : Scope
  Scope2 : Scope
  kWh1 : Display
  MJ : Outport
  kWh : Outport  Port=2
  wires:
  Integrator/1 -> J to MJ/1
  Watt/1 -> Integrator/1
  J to MJ/1 -> Scope1/1, MJ1/1, MJ/1, MJ to kWh/1
  MJ to kWh/1 -> Scope2/1, kWh1/1, kWh/1

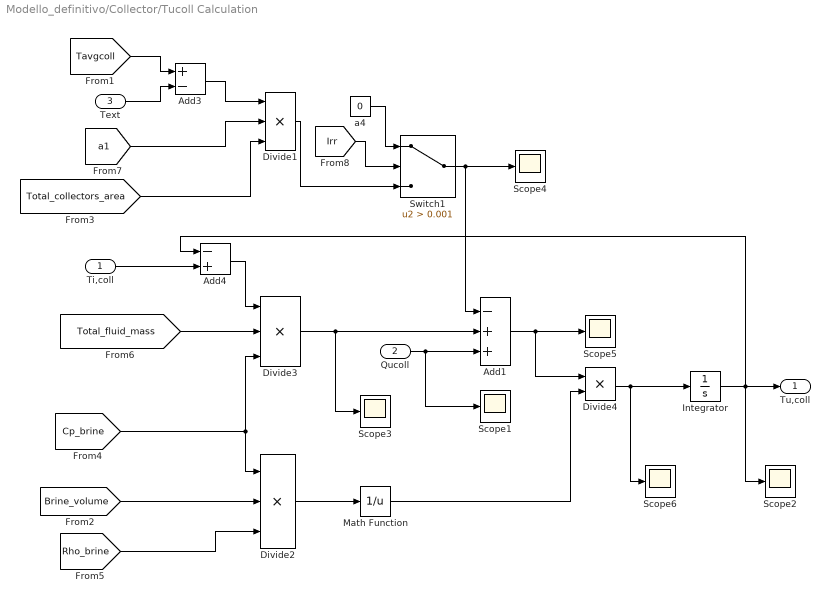
== system Modello_definitivo/Collector/Tucoll Calculation ==
  Ti,coll : Inport
  Qucoll : Inport  Port=2
  Text : Inport  Port=3
  Add1 : Sum  Inputs=-++
  Add3 : Sum  Inputs=+-
  Add4 : Sum  Inputs=-+
  Divide1 : Product  Inputs=***
  Divide2 : Product  Inputs=***
  Divide3 : Product  Inputs=***
  Divide4 : Product  Inputs=**
  Integrator : Integrator  InitialCondition=15
  Math Function : Math  Operator=reciprocal  SaturateOnIntegerOverflow=on
  Scope{1..6} (6 alike) : Scope
  Switch1 : Switch  Criteria=u2 > Threshold  Threshold=0.001
  a4 : Constant  Value=0
  Tu,coll : Outport
  wires:
  [Tavgcoll] -> Add3/1
  Text/1 -> Add3/2
  Add3/1 -> Divide1/1
  [a1] -> Divide1/2
  [Cp_brine] -> Divide2/1, Divide3/3
  [Brine_volume] -> Divide2/2
  [Rho_brine] -> Divide2/3
  Divide2/1 -> Math Function/1
  Ti,coll/1 -> Add4/2
  Divide1/1 -> Switch1/3
  Add4/1 -> Divide3/1
  Divide3/1 -> Add1/2, Scope3/1
  Qucoll/1 -> Add1/3, Scope1/1
  Add1/1 -> Divide4/1, Scope5/1
  Math Function/1 -> Divide4/2
  Divide4/1 -> Integrator/1, Scope6/1
  Integrator/1 -> Tu,coll/1, Scope2/1, Add4/1
  [Total_fluid_mass] -> Divide3/2
  [Total_collectors_area] -> Divide1/3
  [Irr] -> Switch1/2
  a4/1 -> Switch1/1
  Switch1/1 -> Add1/1, Scope4/1

== system Modello_definitivo/Collector/Utility ==
  Add4 : Sum
  Divide1 : Product  Inputs=**
  Divide5 : Product  Inputs=***
  Gain1 : Gain  Gain=1/2  SaturateOnIntegerOverflow=on  OutDataTypeStr=Inherit: Same as input  ParamDataTypeStr=Inherit: Same as input
  Product1 : Product  Inputs=**/  RndMeth=Zero
  contenuto1 : Constant  Value=1000
  tag scope: Brine_volume=global, Tavgcoll=global, Total_collectors_area=global, Total_fluid_mass=global
  wires:
  [Nc] -> Product1/1
  [L] -> Product1/2
  contenuto1/1 -> Product1/3
  Product1/1 -> [Brine_volume]
  [Aap] -> Divide5/3
  [Nc] -> Divide5/2
  [m_brine] -> Divide5/1
  Divide5/1 -> [Total_fluid_mass]
  [Aap] -> Divide1/2
  Divide1/1 -> [Total_collectors_area]
  [Nc] -> Divide1/1
  [Ticoll] -> Add4/1
  [Tucoll] -> Add4/2
  Add4/1 -> Gain1/1
  Gain1/1 -> [Tavgcoll]

== system Modello_definitivo/Pump/Integral Block ==
  Watt : Inport
  Integrator : Integrator
  J to MJ : Gain  Gain=1/1000000
  MJ to kWh : Gain  Gain=1/3.6
  MJ1 : Display
  Scope1 : Scope
  Scope2 : Scope
  kWh1 : Display
  MJ : Outport
  kWh : Outport  Port=2
  wires:
  Integrator/1 -> J to MJ/1
  Watt/1 -> Integrator/1
  J to MJ/1 -> Scope1/1, MJ1/1, MJ/1, MJ to kWh/1
  MJ to kWh/1 -> Scope2/1, kWh1/1, kWh/1

== system Modello_definitivo/Pump/Security System ==
  Tu,pump1 : Inport
  Tu,coll1 : Inport  Port=2
  Add2 : Sum  Inputs=+-
  Add3 : Sum  Inputs=+-
  Relay : Relay  OnSwitchValue=0  OffSwitchValue=-5  OnOutputValue=0  OffOutputValue=1
  Switch : Switch  Criteria=u2 > Threshold  ZeroCross=off
  Switch1 : Switch  Threshold=0.01  ZeroCross=off
  Switch2 : Switch  ZeroCross=off
  Tu,pump : Outport
  wires:
  Tu,coll1/1 -> Switch/3, Switch1/3, Switch2/3
  Tu,pump1/1 -> Switch/1
  Switch/1 -> Switch1/1
  [H] -> Switch1/2
  Switch1/1 -> Switch2/1, Add2/1
  Add2/1 -> Switch2/2
  Switch2/1 -> Tu,pump/1
  [T_s_max] -> Add3/2
  [T3] -> Add3/1, Add2/2
  Add3/1 -> Relay/1
  Relay/1 -> Switch/2

== system Modello_definitivo/Pump/Security System1 ==
  Pump  power1 : Inport
  Add1 : Sum  Inputs=+-
  Add2 : Sum  Inputs=+-
  Constant : Constant  Value=0
  Relay : Relay  OnSwitchValue=0  OffSwitchValue=-5  OnOutputValue=0  OffOutputValue=1
  Scope1 : Scope
  Switch : Switch  Criteria=u2 > Threshold  ZeroCross=off
  Switch1 : Switch  Threshold=0.01  ZeroCross=off
  Pump power : Outport
  wires:
  Constant/1 -> Switch/3, Switch1/3
  [T_s_max] -> Add1/1
  [T3] -> Add1/2
  Pump  power1/1 -> Switch/1
  [H] -> Switch1/2
  Switch/1 -> Switch1/1
  Switch1/1 -> Pump power/1
  [T_s_max] -> Add2/2
  [T3] -> Add2/1
  Add2/1 -> Relay/1
  Relay/1 -> Switch/2, Scope1/1

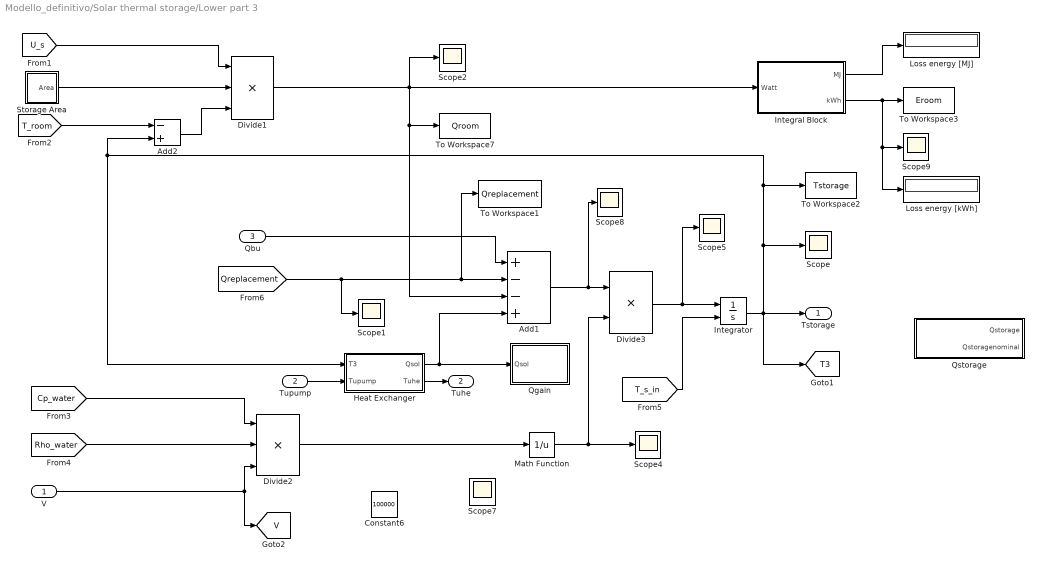
== system Modello_definitivo/Solar thermal storage/Lower part 3 ==
  V : Inport
  Tupump : Inport  Port=2
  Qbu : Inport  Port=3
  Add1 : Sum  Inputs=+--+
  Add2 : Sum  Inputs=-+
  Constant6 : Constant  Value=100000
  Divide1 : Product  Inputs=***
  Divide2 : Product  Inputs=***
  Divide3 : Product  Inputs=**
  Heat Exchanger : Subsystem
  Integral Block : Subsystem
  Integrator : Integrator  InitialConditionSource=external  InitialCondition=T_s_in
  Loss energy [MJ] : Display
      settings: Format=bank
  Loss energy [kWh] : Display
  Math Function : Math  Operator=reciprocal  SaturateOnIntegerOverflow=on
  Qgain : Subsystem
  Qstorage : Subsystem
  Scope{,1..2,4..5,7..9} (8 alike) : Scope
  Storage Area : Subsystem
  To Workspace1 : ToWorkspace  VariableName=Qreplacement  SampleTime=[3600 0]
  To Workspace2 : ToWorkspace  VariableName=Tstorage  SampleTime=[3600 0]
  To Workspace3 : ToWorkspace  VariableName=Eroom  SampleTime=[3600 0]
  To Workspace7 : ToWorkspace  VariableName=Qroom  SampleTime=[3600 0]
  Tstorage : Outport
  Tuhe : Outport  Port=2
  tag scope: T3=global, V=global
  wires:
  [Cp_water] -> Divide2/1
  [U_s] -> Divide1/1
  V/1 -> Divide2/3, [V]
  Divide1/1 -> To Workspace7/1, Add1/3, Integral Block/1(Watt), Scope2/1
  Divide2/1 -> Math Function/1
  Add1/1 -> Divide3/1, Scope8/1
  Math Function/1 -> Divide3/2, Scope4/1
  Divide3/1 -> Integrator/1, Scope5/1
  Integrator/1 -> [T3], Tstorage/1, To Workspace2/1, Heat Exchanger/1(T3), Add2/2, Scope/1
  [Rho_water] -> Divide2/2
  Heat Exchanger/1(Qsol) -> Add1/4, Qgain/1(Qsol)
  [T_room] -> Add2/1
  Heat Exchanger/2(Tuhe) -> Tuhe/1
  Add2/1 -> Divide1/3
  Storage Area/1(Area) -> Divide1/2
  [Qreplacement] -> Scope1/1, To Workspace1/1, Add1/2
  Tupump/1 -> Heat Exchanger/2(Tupump)
  Qbu/1 -> Add1/1
  Integral Block/1(MJ) -> Loss energy [MJ]/1
  Integral Block/2(kWh) -> To Workspace3/1, Scope9/1, Loss energy [kWh]/1
  [T_s_in] -> Integrator/2

== system Modello_definitivo/Subsystem2/Integral Block ==
  Watt : Inport
  Integrator : Integrator
  J to MJ : Gain  Gain=1/1000000
  MJ to kWh : Gain  Gain=1/3.6
  MJ1 : Display
  Scope1 : Scope
  Scope2 : Scope
  kWh1 : Display
  MJ : Outport
  kWh : Outport  Port=2
  wires:
  Integrator/1 -> J to MJ/1
  Watt/1 -> Integrator/1
  J to MJ/1 -> Scope1/1, MJ1/1, MJ/1, MJ to kWh/1
  MJ to kWh/1 -> Scope2/1, kWh1/1, kWh/1

== system Modello_definitivo/Subsystem2/Relazione cons. giornaliero ACS UNI TS 11300-2 (solo per il residenziale) ==
  T_DHW : Inport
  Tacq : Inport  Port=2
  Constant : Constant  Value=0.001162
  FCS1 : Display
  Product1 : Product  Inputs=4  RndMeth=Zero
  Qw,in [Wh/day]2 : Display
  Subtract : Sum  Inputs=+-
  Vw calculation : Subsystem
  Qw,in [Wh/day] : Outport
  Water volume [l/day] : Outport  Port=2
  wires:
  Product1/1 -> Qw,in [Wh/day]/1, Qw,in [Wh/day]2/1
  [S_u] -> Vw calculation/1(Su)
  Subtract/1 -> Product1/3
  Vw calculation/1(Vw) -> Water volume [l/day]/1, Product1/2
  Tacq/1 -> Subtract/2
  Constant/1 -> Product1/1
  [Rho_water] -> Product1/4
  T_DHW/1 -> Subtract/1

== system Modello_definitivo/Back-up/Prova back-up/Controller Qbu ==
  If : If  NumInputs=2  IfExpression=u1>=u2  ZeroCross=off
  If Action Subsystem : Subsystem  TreatAsAtomicUnit=on
  If Action Subsystem3 : Subsystem  TreatAsAtomicUnit=on
  Merge : Merge
  Qbu : Outport
  wires:
  If/1 -> If Action Subsystem/Action
  If Action Subsystem/1(Out1) -> Merge/1
  Merge/1 -> Qbu/1
  If Action Subsystem3/1(Out1) -> Merge/2
  If/2 -> If Action Subsystem3/Action
  [Qstorage] -> If/1
  [Qstoragenominal] -> If/2
  [BU_power] -> If Action Subsystem3/1(In1)

== system Modello_definitivo/Back-up/Prova back-up/Qstored ==
  Add2 : Sum  Inputs=-+
  Product3 : Product  Inputs=***  SaturateOnIntegerOverflow=on  OutDataTypeStr=Inherit: Same as first input
  Qstored : Outport
  wires:
  Product3/1 -> Qstored/1
  [Tacq] -> Add2/1
  [T3] -> Add2/2
  Add2/1 -> Product3/1
  [m] -> Product3/2
  [Cp_water] -> Product3/3

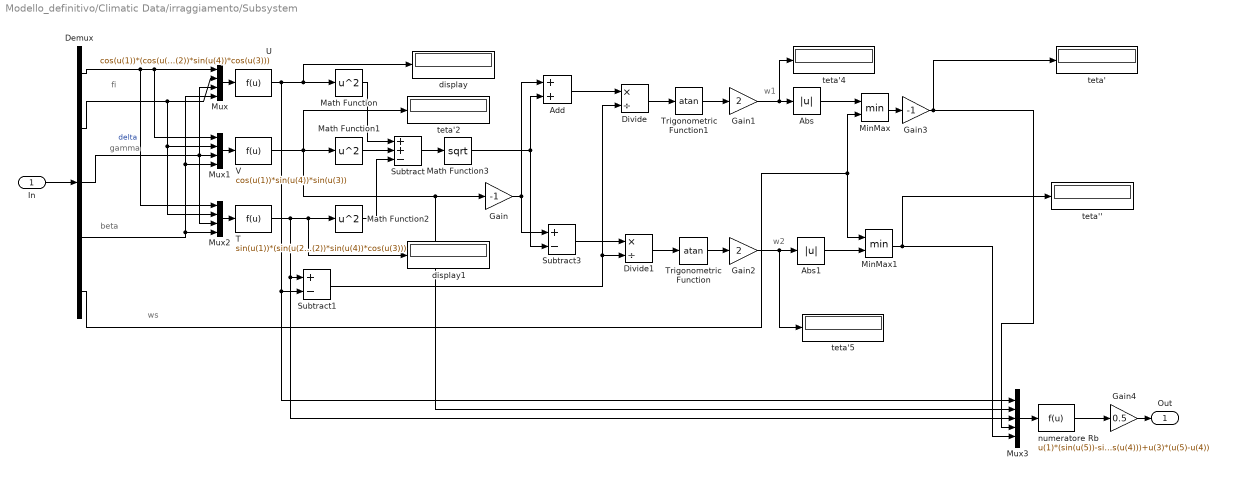
== system Modello_definitivo/Climatic Data/irraggiamento/Subsystem ==
  note: w1
  note: w2
  note: fi
  note: ws
  note: gamma
  note: beta
  In : Inport
  Abs : Abs
  Abs1 : Abs
  Add : Sum
  Demux : Demux  Outputs=5
  Divide : Product  Inputs=*/
  Divide1 : Product  Inputs=*/
  Gain : Gain  Gain=-1
  Gain1 : Gain  Gain=2
  Gain2 : Gain  Gain=2
  Gain3 : Gain  Gain=-1
  Gain4 : Gain  Gain=0.5
  Math Function : Math  Operator=square  SaturateOnIntegerOverflow=on
  Math Function1 : Math  Operator=square  SaturateOnIntegerOverflow=on
  Math Function2 : Math  Operator=square  SaturateOnIntegerOverflow=on
  Math Function3 : Math  Operator=sqrt  SaturateOnIntegerOverflow=on
  MinMax : MinMax  Inputs=2
  MinMax1 : MinMax  Inputs=2
  Mux : Mux
  Mux1 : Mux
  Mux2 : Mux
  Mux3 : Mux  Inputs=5
  Subtract : Sum  Inputs=++-
  Subtract1 : Sum  Inputs=+-
  Subtract3 : Sum  Inputs=+-
  T : Fcn  Expr=sin(u(1))*(sin(u(2))*cos(u(4))-cos(u(2))*sin(u(4))*cos(u(3)))
  Trigonometric Function : Trigonometry  Operator=atan
  Trigonometric Function1 : Trigonometry  Operator=atan
  U : Fcn  Expr=cos(u(1))*(cos(u(2))*cos(u(4))+sin(u(2))*sin(u(4))*cos(u(3)))
  V : Fcn  Expr=cos(u(1))*sin(u(4))*sin(u(3))
  display : Display
  display1 : Display
  numeratore Rb : Fcn  Expr=u(1)*(sin(u(5))-sin(u(4)))-u(2)*(cos(u(5))-cos(u(4)))+u(3)*(u(5)-u(4))
  teta'{,2,4..5} (4 alike) : Display
  teta'' : Display
  Out : Outport
  wires:
  Mux1/1 -> V/1
  Mux/1 -> U/1
  Mux2/1 -> T/1
  Demux/1 -> Mux/1, Mux1/1, Mux2/1  "delta"
  Demux/2 -> Mux/2, Mux1/2, Mux2/2
  T/1 -> Subtract1/1, Mux3/3, Math Function2/1, display1/1
  V/1 -> Math Function1/1, Gain/1, Mux3/2, teta'2/1
  U/1 -> Subtract1/2, Mux3/1, Math Function/1, display/1
  Math Function2/1 -> Subtract/3
  Math Function1/1 -> Subtract/2
  Math Function/1 -> Subtract/1
  Subtract/1 -> Math Function3/1
  Gain/1 -> Subtract3/1, Add/1
  Math Function3/1 -> Add/2, Subtract3/2
  Add/1 -> Divide/1
  Subtract3/1 -> Divide1/1
  Subtract1/1 -> Divide1/2, Divide/2
  Divide/1 -> Trigonometric Function1/1
  Divide1/1 -> Trigonometric Function/1
  Trigonometric Function1/1 -> Gain1/1
  Trigonometric Function/1 -> Gain2/1
  Gain2/1 -> Abs1/1, teta'5/1
  Gain1/1 -> Abs/1, teta'4/1
  Abs/1 -> MinMax/1
  MinMax/1 -> Gain3/1
  Demux/5 -> MinMax/2, MinMax1/1
  Abs1/1 -> MinMax1/2
  Gain3/1 -> teta'/1, Mux3/4
  MinMax1/1 -> teta''/1, Mux3/5
  Mux3/1 -> numeratore Rb/1
  numeratore Rb/1 -> Gain4/1
  Gain4/1 -> Out/1
  In/1 -> Demux/1
  Demux/3 -> Mux/3, Mux1/3, Mux2/3
  Demux/4 -> Mux/4, Mux1/4, Mux2/4

== system Modello_definitivo/Climatic Data/irraggiamento/ws1 ==
  Delta : Inport
  Phi : Inport  Port=2
  Mux1 : Mux  Inputs=2
  Sum : Sum  Inputs=|-+  SaturateOnIntegerOverflow=on
  alba : Display
  cosws : Fcn  Expr=-tan(u[1])*tan(u[2])
  kWh annue2 : Display
  rad grad1 : Fcn  Expr=12-u[1]/15
  rad grad2 : Fcn  Expr=u[1]/pi*180
  rad grad3 : Fcn  Expr=12+u[1]/15
  tramonto : Display
  wsx : Trigonometry  Operator=acos
  Day Length : Outport
  ws : Outport  Port=2
  wires:
  Phi/1 -> Mux1/2
  Delta/1 -> Mux1/1
  rad grad2/1 -> rad grad3/1, rad grad1/1, kWh annue2/1
  wsx/1 -> rad grad2/1, ws/1
  cosws/1 -> wsx/1
  Mux1/1 -> cosws/1
  rad grad1/1 -> alba/1, Sum/1
  rad grad3/1 -> tramonto/1, Sum/2
  Sum/1 -> Day Length/1

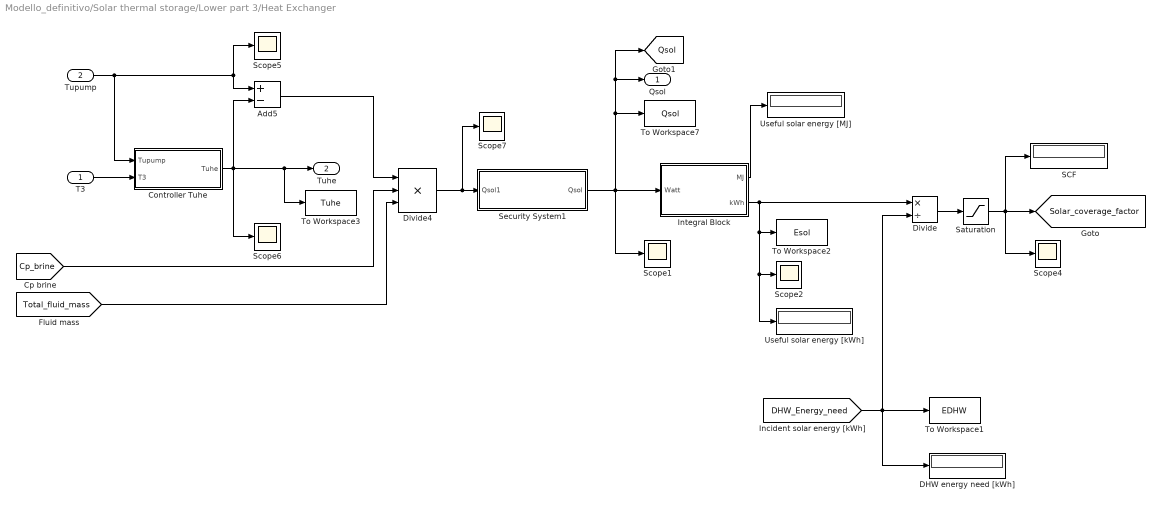
== system Modello_definitivo/Solar thermal storage/Lower part 3/Heat Exchanger ==
  T3 : Inport
  Tupump : Inport  Port=2
  Add5 : Sum  Inputs=+-
  Controller Tuhe : Subsystem
  DHW energy need [kWh] : Display
  Divide : Product  Inputs=*/
  Divide4 : Product  Inputs=***
  Integral Block : Subsystem
  SCF : Display
  Saturation : Saturate  UpperLimit=1  LowerLimit=0
  Scope{1..2,4..7} (6 alike) : Scope
  Security System1 : Subsystem
  To Workspace1 : ToWorkspace  VariableName=EDHW  SampleTime=[3600 0]
  To Workspace2 : ToWorkspace  VariableName=Esol  SampleTime=[3600 0]
  To Workspace3 : ToWorkspace  VariableName=Tuhe  SampleTime=[3600 0]
  To Workspace7 : ToWorkspace  VariableName=Qsol  SampleTime=[3600 0]
  Useful solar energy [MJ] : Display
      settings: Format=bank
  Useful solar energy [kWh] : Display
  Qsol : Outport
  Tuhe : Outport  Port=2
  tag scope: Qsol=global, Solar_coverage_factor=global
  wires:
  Tupump/1 -> Add5/1, Scope5/1, Controller Tuhe/1(Tupump)
  Add5/1 -> Divide4/1
  [Cp_brine] -> Divide4/2
  [Total_fluid_mass] -> Divide4/3
  Divide/1 -> Saturation/1
  Saturation/1 -> Scope4/1, SCF/1, [Solar_coverage_factor]
  Security System1/1(Qsol) -> Integral Block/1(Watt), To Workspace7/1, Qsol/1, [Qsol], Scope1/1
  Divide4/1 -> Security System1/1(Qsol1), Scope7/1
  T3/1 -> Controller Tuhe/2(T3)
  Controller Tuhe/1(Tuhe) -> Add5/2, Scope6/1, Tuhe/1, To Workspace3/1
  Integral Block/1(MJ) -> Useful solar energy [MJ]/1
  Integral Block/2(kWh) -> Divide/1, To Workspace2/1, Scope2/1, Useful solar energy [kWh]/1
  [DHW_Energy_need] -> Divide/2, To Workspace1/1, DHW energy need [kWh]/1

== system Modello_definitivo/Solar thermal storage/Lower part 3/Integral Block ==
  Watt : Inport
  Integrator : Integrator
  J to MJ : Gain  Gain=1/1000000
  MJ to kWh : Gain  Gain=1/3.6
  MJ1 : Display
  Scope1 : Scope
  Scope2 : Scope
  kWh1 : Display
  MJ : Outport
  kWh : Outport  Port=2
  wires:
  Integrator/1 -> J to MJ/1
  Watt/1 -> Integrator/1
  J to MJ/1 -> Scope1/1, MJ1/1, MJ/1, MJ to kWh/1
  MJ to kWh/1 -> Scope2/1, kWh1/1, kWh/1

== system Modello_definitivo/Solar thermal storage/Lower part 3/Qgain ==
  Qsol : Inport
  Controller Qgain : Subsystem
  DHW energy need [kWh] : Display
  Divide : Product  Inputs=/*
  Gained energy [MJ] : Display
      settings: Format=bank
  Gained energy [kWh] : Display
  Integral Block : Subsystem
  SCF : Display
  Saturation : Saturate  UpperLimit=1  LowerLimit=0
  Scope1 : Scope
  Scope4 : Scope
  Scope5 : Scope
  To Workspace1 : ToWorkspace  VariableName=Qgain  SampleTime=[3600 0]
  To Workspace3 : ToWorkspace  VariableName=Egain  SampleTime=[3600 0]
  wires:
  Divide/1 -> Saturation/1
  Saturation/1 -> Scope4/1, SCF/1
  [DHW_Energy_need] -> Divide/1, DHW energy need [kWh]/1
  [Qwhr] -> Controller Qgain/1(Qwhr)
  Controller Qgain/1(Qgain) -> To Workspace1/1, Scope1/1, Integral Block/1(Watt)
  Integral Block/1(MJ) -> Gained energy [MJ]/1
  Integral Block/2(kWh) -> Divide/2, To Workspace3/1, Scope5/1, Gained energy [kWh]/1
  Qsol/1 -> Controller Qgain/2(Qsol)

== system Modello_definitivo/Solar thermal storage/Lower part 3/Qstorage ==
  Add1 : Sum  Inputs=-+
  Add2 : Sum  Inputs=-+
  Gain : Gain  Gain=1/3600
  Gain1 : Gain  Gain=1/3600
  Gained energy [kWh]1 : Display
  Gained energy [kWh]2 : Display
  Product1 : Product  Inputs=****  SaturateOnIntegerOverflow=on  OutDataTypeStr=Inherit: Same as first input
  Product3 : Product  Inputs=****  SaturateOnIntegerOverflow=on  OutDataTypeStr=Inherit: Same as first input
  Scope1 : Scope
  Scope2 : Scope
  Qstorage : Outport
  Qstoragenominal : Outport  Port=2
  tag scope: Qstorage=global, Qstoragenominal=global
  wires:
  [T_acq] -> Add2/1
  [T3] -> Add2/2
  Add2/1 -> Product3/1
  [Rho_water] -> Product3/2
  [Cp_water] -> Product3/3
  [V] -> Product3/4
  Product3/1 -> Gain/1
  Gain/1 -> Qstorage/1, Scope1/1, Gained energy [kWh]1/1, [Qstorage]
  [T_acq] -> Add1/1
  [T_DHW] -> Add1/2
  Add1/1 -> Product1/1
  [Rho_water] -> Product1/2
  [Cp_water] -> Product1/3
  [V] -> Product1/4
  Product1/1 -> Gain1/1
  Gain1/1 -> Qstoragenominal/1, Scope2/1, Gained energy [kWh]2/1, [Qstoragenominal]

== system Modello_definitivo/Solar thermal storage/Lower part 3/Storage Area ==
  Add1 : Sum
  Area1 : Display
  Constant : Constant  Value=0.5
  Divide1 : Product  Inputs=***
  Divide2 : Product  Inputs=***
  Math Function : Math  Operator=square  SaturateOnIntegerOverflow=on
  pi : Constant  Value=pi
  Area : Outport
  wires:
  Add1/1 -> Area/1, Area1/1
  [H_s] -> Divide1/1
  pi/1 -> Divide1/2, Divide2/2
  [D_s] -> Divide1/3, Math Function/1
  Math Function/1 -> Divide2/1
  Constant/1 -> Divide2/3
  Divide1/1 -> Add1/1
  Divide2/1 -> Add1/2

== system Modello_definitivo/Subsystem2/Relazione cons. giornaliero ACS UNI TS 11300-2 (solo per il residenziale)/Vw calculation ==
  Su : Inport
  Display4 : Display
  If : If  IfExpression=u1 <= 35  ElseIfExpressions=u1<=50, u1<=200
  If Action Subsystem : Subsystem  TreatAsAtomicUnit=on
  If Action Subsystem1 : Subsystem  TreatAsAtomicUnit=on
  If Action Subsystem2 : Subsystem  TreatAsAtomicUnit=on
  If Action Subsystem3 : Subsystem  TreatAsAtomicUnit=on
  Merge : Merge  Inputs=4
  Vw : Outport
  wires:
  If/1 -> If Action Subsystem/Action
  Su/1 -> If/1, If Action Subsystem/1(Su), If Action Subsystem1/1(Su), If Action Subsystem2/1(Su), If Action Subsystem3/1(Su)
  If/2 -> If Action Subsystem1/Action
  If/3 -> If Action Subsystem2/Action
  If/4 -> If Action Subsystem3/Action
  If Action Subsystem/1(Water Volume) -> Merge/1
  If Action Subsystem1/1(Water Volume) -> Merge/2
  If Action Subsystem2/1(Water Volume) -> Merge/3
  If Action Subsystem3/1(Water Volume) -> Merge/4
  Merge/1 -> Vw/1, Display4/1

== system Modello_definitivo/Back-up/Prova back-up/Controller Qbu/If Action Subsystem ==
  Action Port : ActionPort  ActionType=then
  Constant : Constant  Value=0
  Out1 : Outport
  wires:
  Constant/1 -> Out1/1

== system Modello_definitivo/Back-up/Prova back-up/Controller Qbu/If Action Subsystem3 ==
  In1 : Inport
  Action Port : ActionPort  ActionType=else
  Out1 : Outport
  wires:
  In1/1 -> Out1/1

== system Modello_definitivo/Solar thermal storage/Lower part 3/Heat Exchanger/Controller Tuhe ==
  Tupump : Inport
  T3 : Inport  Port=2
  Add1 : Sum
  Add4 : Sum  Inputs=+-
  Divide1 : Product  Inputs=**
  Fcn : Fcn  Expr=exp((-u[1])/(u[2]*u[3]))
  Mux : Mux  Inputs=3
  Scope1 : Scope
  Scope2 : Scope
  Scope8 : Scope
  Switch1 : Switch  Criteria=u2 > Threshold  ZeroCross=off
  Tuhe : Outport
  wires:
  Tupump/1 -> Add4/1, Scope2/1
  [Total_fluid_mass] -> Mux/3
  Mux/1 -> Fcn/1
  Add4/1 -> Divide1/1
  Fcn/1 -> Divide1/2
  Divide1/1 -> Add1/2, Scope8/1
  T3/1 -> Add4/2, Add1/1
  Add1/1 -> Switch1/1
  Switch1/1 -> Tuhe/1, Scope1/1
  [Pelpump] -> Switch1/2
  [Tucoll] -> Switch1/3
  [UA_s_ex] -> Mux/1
  [Cp_brine] -> Mux/2

== system Modello_definitivo/Solar thermal storage/Lower part 3/Heat Exchanger/Integral Block ==
  Watt : Inport
  Integrator : Integrator
  J to MJ : Gain  Gain=1/1000000
  MJ to kWh : Gain  Gain=1/3.6
  MJ1 : Display
  Scope1 : Scope
  Scope2 : Scope
  kWh1 : Display
  MJ : Outport
  kWh : Outport  Port=2
  wires:
  Integrator/1 -> J to MJ/1
  Watt/1 -> Integrator/1
  J to MJ/1 -> Scope1/1, MJ1/1, MJ/1, MJ to kWh/1
  MJ to kWh/1 -> Scope2/1, kWh1/1, kWh/1

== system Modello_definitivo/Solar thermal storage/Lower part 3/Heat Exchanger/Security System1 ==
  Qsol1 : Inport
  Add1 : Sum  Inputs=+-
  Add2 : Sum  Inputs=+-
  Constant : Constant  Value=0
  Switch : Switch  Criteria=u2 > Threshold  ZeroCross=off
  Switch1 : Switch  Criteria=u2 > Threshold  ZeroCross=off
  Qsol : Outport
  wires:
  Add1/1 -> Switch/2
  Constant/1 -> Switch/3, Switch1/3
  [T_s_max] -> Add1/1
  [T3] -> Add1/2
  Qsol1/1 -> Switch/1
  [Tupump] -> Add2/1
  [T3] -> Add2/2
  Add2/1 -> Switch1/2
  Switch/1 -> Switch1/1
  Switch1/1 -> Qsol/1

== system Modello_definitivo/Solar thermal storage/Lower part 3/Qgain/Controller Qgain ==
  Qwhr : Inport
  Qsol : Inport  Port=2
  If : If  NumInputs=2  IfExpression=u2<0  ElseIfExpressions=u2>=u1,u2<u1  ShowElse=off  ZeroCross=off
  If Action Subsystem : Subsystem  TreatAsAtomicUnit=on
  If Action Subsystem1 : Subsystem  TreatAsAtomicUnit=on
  If Action Subsystem3 : Subsystem  TreatAsAtomicUnit=on
  Merge : Merge  Inputs=3
  Qstored : Subsystem
  Qgain : Outport
  wires:
  Qwhr/1 -> If/1, If Action Subsystem1/1(In1)
  If/1 -> If Action Subsystem/Action
  If Action Subsystem/1(Out1) -> Merge/1
  If Action Subsystem1/1(Out1) -> Merge/2
  If Action Subsystem3/1(Out1) -> Merge/3
  If/2 -> If Action Subsystem1/Action
  If/3 -> If Action Subsystem3/Action
  Qstored/1(Qstored) -> If/2, If Action Subsystem3/1(In1)
  Qsol/1 -> Qgain/1

== system Modello_definitivo/Solar thermal storage/Lower part 3/Qgain/Integral Block ==
  Watt : Inport
  Integrator : Integrator
  J to MJ : Gain  Gain=1/1000000
  MJ to kWh : Gain  Gain=1/3.6
  MJ1 : Display
  Scope1 : Scope
  Scope2 : Scope
  kWh1 : Display
  MJ : Outport
  kWh : Outport  Port=2
  wires:
  Integrator/1 -> J to MJ/1
  Watt/1 -> Integrator/1
  J to MJ/1 -> Scope1/1, MJ1/1, MJ/1, MJ to kWh/1
  MJ to kWh/1 -> Scope2/1, kWh1/1, kWh/1

== system Modello_definitivo/Subsystem2/Relazione cons. giornaliero ACS UNI TS 11300-2 (solo per il residenziale)/Vw calculation/If Action Subsystem ==
  Su : Inport
  Action Port : ActionPort  ActionType=then
  Add : Sum
  Product : Product  RndMeth=Zero
  a : Constant  Value=0
  b : Constant  Value=50
  Water Volume : Outport
  wires:
  Su/1 -> Product/1
  a/1 -> Product/2
  Product/1 -> Add/1
  b/1 -> Add/2
  Add/1 -> Water Volume/1

== system Modello_definitivo/Subsystem2/Relazione cons. giornaliero ACS UNI TS 11300-2 (solo per il residenziale)/Vw calculation/If Action Subsystem1 ==
  Su : Inport
  Action Port : ActionPort  ActionType=elseif
  Add : Sum
  Product : Product  RndMeth=Zero
  a : Constant  Value=2.667
  b : Constant  Value=-43.33
  Water Volume : Outport
  wires:
  Su/1 -> Product/1
  a/1 -> Product/2
  Product/1 -> Add/1
  b/1 -> Add/2
  Add/1 -> Water Volume/1

== system Modello_definitivo/Subsystem2/Relazione cons. giornaliero ACS UNI TS 11300-2 (solo per il residenziale)/Vw calculation/If Action Subsystem2 ==
  Su : Inport
  Action Port : ActionPort  ActionType=elseif
  Add : Sum
  Product : Product  RndMeth=Zero
  a : Constant  Value=1.067
  b : Constant  Value=36.67
  Water Volume : Outport
  wires:
  Su/1 -> Product/1
  a/1 -> Product/2
  Product/1 -> Add/1
  b/1 -> Add/2
  Add/1 -> Water Volume/1

== system Modello_definitivo/Subsystem2/Relazione cons. giornaliero ACS UNI TS 11300-2 (solo per il residenziale)/Vw calculation/If Action Subsystem3 ==
  Su : Inport
  Action Port : ActionPort  ActionType=else
  Add : Sum
  Product : Product  RndMeth=Zero
  a : Constant  Value=0
  b : Constant  Value=250
  Water Volume : Outport
  wires:
  Su/1 -> Product/1
  a/1 -> Product/2
  Product/1 -> Add/1
  b/1 -> Add/2
  Add/1 -> Water Volume/1
